simulink library "Mylibrary"  (Simulink 8.3)
settings: Solver=ode45  StartTime=0.0  StopTime=10.0  RelTol=1e-3
undefined symbols (not defined in the file or in its folder): Delay, epsilon, L, Mode, R, T_Trigger, tau_bar, Ts, Ts1, vd, Vehicle_Index, vp, x0, y0
undefined symbols (not defined in the file): d1, m1, psi20, Vx, Vy, x20, y20
libraries: Mylibrary x3
(part 2 of 3)

== matlab function Virtual Target Lapier/Virtual Target Position 2 ==
  settings: updateMethod=DISCRETE  sampleTime=0.2
  data: gamma_c output double; gamma input double size=1; pd output double; vd_bar output double size=1; theta_c output double size=1; vd input double; L input double; R input double; d input double; m input double
function [gamma_c,pd,vd_bar,theta_c] = fcn(gamma,vd,L,R,d,m) 
s1=L-m;
s2=s1+pi*(R-d);
s3=s2+L;
s4=s3+pi*(R+d);
s5=s4+m;
ratio1=(R-d)/R;
ratio2=(R+d)/R;
ratio1=1;
ratio2=1;
if gamma<s5;
    cycle=0;
else
    cycle=1;
end

s=gamma-s5*cycle;

if s<s1                                    % first segment of straight line;
    vd_bar=vd;
    xd=0+d;
    yd=s+R+m;
    theta_c=90;
    gamma_c=s+s5*cycle;                                  % the segment is parallel with x
elseif (s>=s1) && (s<=s2)                  % second segment, a circumference 
    vd_bar=ratio1*vd;
    theta_c=90-(s-s1)*180/((R-d)*pi);
    xd=d+(R-d)*(1-sind(theta_c));
    yd=L+R+(R-d)*cosd(theta_c);   
    gamma_c=s1+(s-s1)*R/(R-d)+s5*cycle; 
elseif (s>s2) && (s<=s3)                   % third segment, a straight line 
    vd_bar=vd;
    yd=s3-s+R;  
    theta_c=-90;
    xd=d+2*(R-d);
    gamma_c=s+d*pi+s5*cycle;
elseif (s>s3) && (s<=s4)   
    vd_bar=ratio2*vd;
    theta_c=-90+(s-s3)/(R+d);
    xd=d+2*(R-d)+(R+d)*(1+sin(theta_c));
    yd=R-(R+d)*cos(theta_c);
    gamma_c=s3+d*pi+(s-s3)*R/(R+d)+s5*cycle;   
else
    vd_bar=vd;
    yd=(s-s4)+R;
    xd=d+4*R;
    theta_c=90;
    gamma_c=s+s5*cycle;
end

if cycle ==0
pd=[xd;cycle*4*R+yd];    
else 
pd=[xd;cycle*4*R+yd];
end

== matlab function Simplified Estimator of Gamma for two vehicle/Estimator ==
  data: vd_t output double size=1; DataToTran output double size=2; gamma_c input double; gamma_c_M input double; t input double; Re_Data1 input double size=2; Re_Data2 input double; Com_Sig input double; gamma_hat output double; tau_bar input double; Mode input double; vd input double; e_int input double; e output double; e_int_event output double
function [vd_t,DataToTran,gamma_hat,e,e_int_event] = fcn(gamma_c,gamma_c_M,t,Re_Data1,Re_Data2,Com_Sig,tau_bar,Mode,vd,e_int)

%% 
kg=1;
% L=[1 -1;
%    -1 1]; 

%% Reset estimator of gamma
persistent gamma_cn1 gamma_cn2 gamma_c0 tc1 tc2 tcn11 tcn12 tcn21 tcn22 tem_c tem_cn1 tem_cn2 reset_c reset_cn1 reset_cn2 e_int_t;   
if isempty(gamma_cn1)
    gamma_cn1=0;
    gamma_cn2=0;
    gamma_c0=0;
    tcn11=t;
    tcn12=t;
    tcn21=t;
    tcn22=t;
    tc1=t;
    tc2=t;
    tem_c=t;
    tem_cn1=t;
    tem_cn2=t;
    reset_c=false;
    reset_cn1=false;
    reset_cn2=false;
    e_int_t=0;
end
%% Reset estimator for gamma_c of first neighbor;
if (Re_Data1(1)~=0)                                  % If recived new data, reset estimator that the current vehicle thinks about the neighbor vehicle
    tcn11=Re_Data1(1); 
    tem_cn1=Re_Data1(2);
    reset_cn1=true;
end   
if (t-tcn11>tau_bar)&&reset_cn1
    gamma_cn1=tem_cn1+vd*tau_bar;
    reset_cn1=false;
    tcn12=t;
end
%% Reset estimator for gamma_c of second neighbor;
if (Re_Data2(1)~=0)                                  % If recived new data, reset estimator that the current vehicle thinks about the neighbor vehicle
    tcn21=Re_Data1(1); 
    tem_cn2=Re_Data2(2);
    reset_cn2=true;
end   
if (t-tcn21>tau_bar)&&reset_cn2
    gamma_cn2=tem_cn2+vd*tau_bar;
    reset_cn2=false;
    tcn22=t;
end
%% Reset estimator for gamma_c of current vehicle   % When it sends its coordinate state to neighbor, it needs to update its estimator too to synchoronize with the neighbor
if (Com_Sig~=0)
    tc1=t;
    tem_c=gamma_c;
    reset_c=true;
end
if (t-tc1>tau_bar)&& reset_c
    gamma_c0=tem_c+vd*tau_bar;
    reset_c=false;
    tc2=t;
end
%% Run estimators
gamma_c_hat=gamma_c0+vd*(t-tc2);
gamma_c_n1_hat=gamma_cn1+vd*(t-tcn12);
gamma_c_n2_hat=gamma_cn2+vd*(t-tcn22);

gamma_hat=[gamma_c_hat;gamma_c_n1_hat;gamma_c_n2_hat]; 

ki=.1;
if Mode==0
     e=gamma_c_M-0.5*(Re_Data1(2)+Re_Data2(2));
elseif Mode==1
    if (Re_Data1(2)~=0)
       e=gamma_c_M-0.5*(Re_Data1(2)+Re_Data2(2));
    else   
       e=0;
    end
else
    if (Re_Data1(2)~=0) 
       e=gamma_c_M-Re_Data1(2);
       e_int_t=e_int_t+e;
    else
        e=0;
    end
     if (Re_Data2(2)~=0) 
       e=gamma_c_M-Re_Data2(2);
       e_int_t=e_int_t+e;
     else
         e=0;
     end
end
%% Compute correction term 
if Mode==0;                                     % if Mode==0, continous communication, we use direct data recieved from neighbor.
    vd_t=-kg*e-ki*e_int; 
elseif Mode==1
    e1=(gamma_c-0.5*(gamma_c_n1_hat+gamma_c_n2_hat));
    vd_t=-kg*e1-ki*e_int;
else
    e1=(gamma_c-0.5*(gamma_c_n1_hat+gamma_c_n2_hat));
    vd_t=-kg*e1-ki*e_int_t;
end
e_int_event=e_int_t;
%% Prepare Data for transmition block
gamma_e=gamma_c-gamma_c_hat;
% DataToTran=[gamma_c;gamma_e;gamma_hat];
DataToTran=[gamma_c;gamma_e];

== matlab function Medusa_Model/State Derivatives ==
  data: x input double; y input double; yaw input double; u input double; v input double; r input double; tau_u input double; dot_x output double; tau_r input double; dot_y output double; dot_yaw output double; dot_u output double; dot_v output double; dot_r output double; fu input double; fv input double; fr input double; Vcx input double; Vcy input double
function [dot_x,dot_y,dot_yaw,dot_u,dot_v,dot_r] = fcn(x,y,yaw,u,v,r,tau_u,tau_r,fu,fv,fr, Vcx, Vcy)
% This is model of Sirene given in the thesis of Vanni

mass = 17.0;
I_z = 1;
X_dot_u = -20;
Y_dot_v = -30;%-1.3175;
N_dot_r = -8.69;% -0.5;
X_u = -0.2;
Y_v = -50;
N_r = -4.14; %-0.1
X_uu = -25; 
Y_vv = -0.01;%-101.2776;
N_rr = -6.23; %-21

%%%%%% masses
m_u = mass - X_dot_u;
m_v = mass - Y_dot_v;
m_r = I_z - N_dot_r;
m_uv = m_u - m_v;

%%%%%%%%% drag

d_u = -X_u - X_uu*abs(u);
d_v = -Y_v - Y_vv*abs(v);
d_r = -N_r - N_rr*abs(r);

%%%%%%%%% Dynamics

dot_u = 1/m_u*(tau_u + m_v*v*r - d_u*u+fu);
dot_v = 1/m_v*(-m_u*u*r - d_v*v+fv);
dot_r = 1/m_r*(tau_r + m_uv*u*v - d_r*r+fr);

dot_x = u*cos(yaw) - v*sin(yaw) + Vcx;
dot_y = u*sin(yaw) + v*cos(yaw) + Vcy;
dot_yaw = r;

== matlab function PF Controller+Medusa/Path Following Controller/Inner-loop controller ==
  settings: sampleTime=Ts
  data: ud_dot input double; ud input double size=2; ur input double; r input double; tau_r output double; tau_u output double; vr_hat input double
function [tau_r,tau_u]  = fcn(ud_dot,ud,ur,r,vr_hat)
%#codegen                        % design speed profile
u=[ur;r];
% Vcxy=[0;0];                       % without constant current in inertial frame
% Vc_hat=R'*Vcxy; 


mass = 17.0;
I_z = 1;
X_dot_u = -20;
Y_dot_v = -30;%-1.3175;
N_dot_r = -8.69;% -0.5;
X_u = -0.2;
N_r = -4.14; %-0.1
X_uu = -25; 
N_rr = -6.23; %-21


dur = -X_u - X_uu*abs(ur);
dr = -N_r - N_rr*abs(r);
D=[dur 0;
    0  dr];

m_u = mass - X_dot_u;
m_v = mass - Y_dot_v;

mr = I_z - N_dot_r;


muv=m_u-m_v;
C=[0 -m_v*vr_hat;
    -muv*vr_hat 0];
M=[m_u 0;
    0 mr];

%% Innerloop controller
    ku=100;kr=10;
    Kd=[ku 0; 
        0 kr];
%     ud_dot=[0;0];
    tau=-Kd*(u-ud)+D*ud+C*u+M*ud_dot;
%% Apply torque and force to vehicles
    tau_u=tau(1);
    tau_r=tau(2);

== matlab function PF Controller+Medusa/Path Following Controller/Observer/observer of current and vr  ==
  settings: sampleTime=Ts
  data: vr_hat_old input double; ur input double; psi input double; p input double size=2; Vcxy_hat_old input double; p_hat_old input double; vr_hat output double; Vc_hat output double; Vcxy_hat output double; p_hat output double; r input double
function [vr_hat,Vc_hat,Vcxy_hat,p_hat]  = Current_obs(vr_hat_old,ur,psi,p,Vcxy_hat_old,p_hat_old,r)
Ts=0.2;
R=[cos(psi)   -sin(psi);
   sin(psi)    cos(psi)]; 
p_t=p-p_hat_old;
Vr=[ur;vr_hat_old];

%% current observer

Kp=10*[1 0;
       0 1];
Kc=10*[1 0;
      0 1];
p_hat=p_hat_old+Ts*(R*Vr+Vcxy_hat_old+Kp*p_t);
Vcxy_hat=Vcxy_hat_old+Ts*Kc*p_t;
%% estimation of vr
mass = 17.0;

X_dot_u = -20;
Y_dot_v = -30;%-1.3175;


Y_v = -50;

Y_vv = -0.01;%-101.2776;
  
  m_u = mass - X_dot_u;
  m_v = mass - Y_dot_v;
  d_v = -Y_v - Y_vv*abs(vr_hat_old);
  
  vr_hat=vr_hat_old+Ts*(-m_u*ur*r/m_v-d_v*vr_hat_old/m_v);
%% Transform the coodinates of current to body frame
Vc_hat=R'*Vcxy_hat;

== matlab function gamma estimator single neighbor/Estimator ==
  data: t input double; Re_Data input double; gamma_dot output double; gamma_c input double; trigger output double; x0 output double; tau_bar input double; Vehicle_Index input double; gamma_hat input double size=2; vd_t output double; DataToTran output double size=4; Mode input double; Com_Sig input double
function [gamma_dot,trigger,x0,vd_t,DataToTran] = fcn(t,Re_Data,gamma_c,tau_bar,Vehicle_Index,gamma_hat,Mode,Com_Sig)

%% compute error term of velocity 
% kg=0.3;
vd=1;kg=0.05;
L=[1 -1;
   -1 1]; 
% trigger=Re_Data(2); 
% x0=[gamma_c;Re_Data(2)];
% gamma_dot = vd*[1;1];

%% Reset estimator of gamma
persistent data_old t_recieve trigger_tem gamma_n;   
if isempty(data_old)
    data_old=Re_Data(1);
    t_recieve=t;
    trigger_tem=0;
    gamma_n=0;
end
if (Re_Data(1)~=0)
    t_recieve=Re_Data(1);
    trigger_tem=0;
    gamma_n=Re_Data(2)+vd*tau_bar;
end 
if (t-t_recieve>tau_bar)
    trigger_tem=1;
end
data_old=Re_Data(1);


x0=[gamma_c;gamma_n];
trigger=trigger_tem;
% gamma_dot = vd*[1;1]-kg*L*gamma_hat;
gamma_dot = vd*[1;1];

%% Compute correction term 
if Mode==0;
    gamma_c_n_hat=Re_Data(2);
else
    gamma_c_n_hat=gamma_hat(2);
end
% gamma_c_hat=gamma_hat(Vehicle_Index);
vd_t=-kg*(gamma_c-gamma_c_n_hat);  
%% Prepare Data for transmition block
gamma_e=gamma_c-gamma_hat(1);
DataToTran=[gamma_c;gamma_e;gamma_hat];

== matlab function PF Controller+Medusa/Path Following Controller/Outer-loop controller ==
  settings: updateMethod=CONTINUOUS  sampleTime=Ts
  data: gamma_dot input double size=1; gamma_ddot output double size=1; pd input double size=2; pd_gamma input double size=2; vd_bar input double; p input double size=2; psi input double; Vc_hat input double size=2; ud output double size=2; vr_hat input double; vd_t input double
function [gamma_ddot,ud]  = fcn(gamma_dot,pd,pd_gamma,vd_bar,p,psi,Vc_hat,vr_hat,vd_t)
%#codegen                        % design speed profile
vd=vd_bar+vd_t;
%% put constraint for vd

%%
R=[cos(psi)   -sin(psi);
   sin(psi)    cos(psi)]; 
e=R'*(p-pd);
% Vcxy=[0;0];                       % without constant current in inertial frame
% Vc_hat=R'*Vcxy; 
%% Outerloop controller
    delta=-0.2;
    Delta_inv= [1    0;
                0 -1/delta]; 
    %     kx=1; ky=0.6;    
    kx=1; ky=0.6;   
    Kk=[kx 0;
        0  ky];
    ud=Delta_inv*(-Kk*tanh(e-[delta;0])-[0;vr_hat]-Vc_hat+R'*pd_gamma*vd);
    
    %
% ud_max=1.5;
% ud_min=-1;
%     
% if ud(1)>=ud_max
%     ud(1)=ud_max;
% elseif ud(1)<=ud_min
%     ud(1)=ud_min;
% end
       
 %% control gamma   
%     kz=100;
    kz=30;
    vd_dot=0;
    gamma_ddot=-kz*(gamma_dot-vd_bar)+vd_dot+(e-[delta;0])'*R'*pd_gamma + kz*vd_t;  % not that, vd=constant => vd_partial=0 => z=gamma_dot
    %gamma_ddot=0;

== matlab function  Real MEDUSA Vehicle (2013)/Medusa/Dynamics1/State Derivatives ==
  data: x input double; y input double; yaw input double; u input double; v input double; r input double; tau_u input double; dot_x output double; tau_r input double; dot_y output double; dot_yaw output double; dot_u output double; dot_v output double; dot_r output double; fu input double; fv input double; fr input double; Vcx input double; Vcy input double
function [dot_x,dot_y,dot_yaw,dot_u,dot_v,dot_r] = fcn(x,y,yaw,u,v,r,tau_u,tau_r,fu,fv,fr, Vcx, Vcy)
%state = [x, y, yaw, u, v, r]

% %%%%%% Coefficients
% mass = 17.0;
% I_z = 4.14;
% X_dot_u = -20;
% Y_dot_v = -1.3175;
% N_dot_r =  -8.69;
% X_u = -0.2;
% Y_v = -55.117;
% N_r = -4.14;
% X_uu = -25; 
% Y_vv = -101.2776;
% N_rr = -6.23;

%%%%%% Coefficients
mass = 17.0;
I_z = 1;
X_dot_u = -20;
Y_dot_v = -30;%-1.3175;
N_dot_r = -8.69;% -0.5;
X_u = -0.2;
Y_v = -50;
N_r = -4.14; %-0.1
X_uu = -25; 
Y_vv = -0.01;%-101.2776;
N_rr = -6.23; %-21

%%%%%% masses
m_u = mass - X_dot_u;
m_v = mass - Y_dot_v;
m_r = I_z - N_dot_r;
m_uv = m_u - m_v;

%%%%%%%%% drag

d_u = -X_u - X_uu*abs(u);
d_v = -Y_v - Y_vv*abs(v);
d_r = -N_r - N_rr*abs(r);

%%%%%%%%% Dynamics

dot_u = 1/m_u*(tau_u + m_v*v*r - d_u*u+fu);
dot_v = 1/m_v*(-m_u*u*r - d_v*v+fv);
dot_r = 1/m_r*(tau_r + m_uv*u*v - d_r*r+fr);

dot_x = u*cos(yaw) - v*sin(yaw) + Vcx;
dot_y = u*sin(yaw) + v*cos(yaw) + Vcy;
dot_yaw = r;

== matlab function  Real MEDUSA Vehicle (2013)/Medusa/Heading Controller/Embedded MATLAB Function1 ==
  data: YawRef input double; x output double; Yaw input double; Yawrate input double; Kd parameter double; Kp parameter double
function x = controller(YawRef, Yaw, Yawrate, Kd, Kp)
err = ( YawRef- Yaw );
if(err>180) 
     err=err-360;
elseif(err<-180) 
     err=360+err;
end

x=Kp*err-Kd*Yawrate;

== matlab function  Real MEDUSA Vehicle (2013)/Medusa/MotorPower/Embedded MATLAB Function ==
  data: Sm output double; Pm output double; Cm_Speed input double; Dm_Head input double; Cm input double; Dm input double; InnerLoops input double
function [Sm,Pm] = fcn(Cm_Speed, Dm_Head, Cm, Dm, InnerLoops)
Cm_sqr=0;
Dm_sqr=0;
% switch InnerLoops
%     case 0
%         ; % Don't do anything
%     case 1
%         Cm_sqr=Cm_Speed;
%         Dm_sqr=Dm_Head;
%     case 2
%         Cm_sqr=Cm*abs(Cm);
%         Dm_sqr=Dm_Head;
%     case 3
%         Cm_sqr=Cm_Speed;
%         Dm_sqr=Dm*abs(Dm);
%     case 4
        Cm_sqr=Cm*abs(Cm);
        Dm_sqr=Dm*abs(Dm);
%     otherwise
% end

Pm = round(sqrt(abs(Cm_sqr+Dm_sqr))*sign(Cm_sqr+Dm_sqr));
Sm = round(sqrt(abs(Cm_sqr-Dm_sqr))*sign(Cm_sqr-Dm_sqr));

== matlab function PF Controller Lapier Miguel Hung  ==
  settings: updateMethod=DISCRETE  sampleTime=0.2
  data: vd_t input double size=1; p input double size=2; r input double; yaw input double size=1; u input double size=1; gamma_c output double size=1; vcxy_hat output double; yaw_ref output double; r_ref output double; precise output double; u_ref output double; pd output double; L parameter double; R parameter double; d parameter double; m parameter double; vd parameter double
function [gamma_c,vcxy_hat,yaw_ref,r_ref,precise,u_ref,pd] = fcn(vd_t,p,r,yaw,u,L, R, d, m, vd)
%% Declare and initialize global variales                                   These variables will be kept in memory during execuation
    Ts=0.2;         
    persistent vr_hat_old   vr_hat    % sampling time
    persistent p_hat_old    p_hat   Vcxy_hat_old Vcxy_hat 
    persistent gamma_old gamma_dot_old
    if isempty(p_hat)
        vr_hat_old=0;            vr_hat=0; 
        p_hat=p;                 p_hat_old=p;    Vcxy_hat_old=[0;0];  Vcxy_hat=[0;0];
        gamma_old=0;  
        gamma_dot_old=0;
    end    
%% Vehicle Prameters
    mass = 17.0;
    X_dot_u = -20;
    Y_dot_v = -30;                                                              %-1.3175;
    Y_v = -50;
    Y_vv = -0.01;                                                               %-101.2776;
    % masses
    m_u = mass - X_dot_u;
    m_v = mass - Y_dot_v;
    N_r = -4.14; %-0.1
    N_rr = -6.23; %-21
%% Update path
    [gamma_c,vd_bar,path_point,s_dot] = path(gamma_old,L, R, d, m, vd);
    theta_c=path_point(3)*180/pi;
    c_c=path_point(5);
    g_c=path_point(6);
    pd=[path_point(1);path_point(2)];
%% error between vehicle and rabbit
   R1=[cosd(theta_c)       sind(theta_c);     % From {I} to {F}
      -sind(theta_c)       cosd(theta_c)]; 
   e=p-pd;
   e_f=R1*e;
   s1=e_f(1);
   y1=e_f(2);      
%% Estimate vr
    d_v = -Y_v - Y_vv*abs(vr_hat);
    vr_hat_dot=-m_u*u*r/m_v-d_v*vr_hat/m_v;
    vr_hat=vr_hat_old+Ts*vr_hat_dot;
    vr_hat_old=vr_hat; 
%% Estimate current 
% Estimate current in Inertial frame
    R2=[cosd(yaw)        -sind(yaw);     % From {B} to {I}
        sind(yaw)         cosd(yaw)]; 
    p_t=p-p_hat;
    Vr=[u;0*vr_hat];
    Kp=10*[1 0;
           0 1];
    Kc=10*[1 0;
          0 1];
    p_hat_dot=R2*Vr+Vcxy_hat+Kp*p_t;
    p_hat=p_hat_old+Ts*p_hat_dot;
    p_hat_old=p_hat;
    Vcxy_hat_dot=Kc*p_t;
    Vcxy_hat=Vcxy_hat_old+Ts*Vcxy_hat_dot;
    Vcxy_hat_old=Vcxy_hat;
    vcxy_hat=Vcxy_hat;
% Transform the estimated current to Frenet frame
    Vc_hat_f=R1*Vcxy_hat;                      
    Vc_par=Vc_hat_f(1);
    Vc_per=Vc_hat_f(2);
%% Outerloop Controller
   s=2;
   a=y1/s+Vc_per/u;
%    a=y1/s;                                             % No current                          
   a= min(max(a, -1), 1);
   theta=-asind(a);
% Yaw reference
   yaw_ref=theta_c+theta;
%    yaw_ref=60;
% Yaw rate reference
    r_ref=-c_c*s_dot*180/pi;
%     r_ref=0;
% speed reference
    u_ref=vd_bar+vd_t;
%% Gamma Controller
   k1=1;
   gamma_dot=u*cosd(yaw-theta_c)+k1*s1+Vc_par;
   s_acc=(gamma_dot-gamma_dot_old)/Ts;
   gamma_dot_old=gamma_dot;
   gamma=gamma_old+Ts*gamma_dot;
   gamma_old=gamma;
% Precicise 
    r_rad=r*pi/180;
    precise=-g_c*s_dot^2-c_c*s_acc - N_r*r_rad - N_rr*r_rad*abs(r_rad);
%     precise=0;
end
function [gamma_c,vd_bar,path_point,s_dot] = path(gamma,L, R, d, m, vd) 
s1=L-m;
s2=s1+pi*(R-d);
s3=s2+L;
s4=s3+pi*(R+d);
s5=s4+m;
ratio1=(R-d)/R;
ratio2=(R+d)/R;
ratio1=1;
ratio2=1;
if gamma<s5;
    cycle=0;
else
    cycle=1;
end
Ts=0.2;
s=gamma-s5*cycle;

persistent c_c_old gamma_old
if isempty(c_c_old)
    c_c_old=0;
    gamma_old=0;
end

if s<s1                                    % first segment of straight line;
    vd_bar=vd;
    xd=0+d;
    yd=s+R+m;
    theta_c=pi/2;
    gamma_c=s+s5*cycle;                    % the segment is parallel with x
    c_c=0;
    c_c_dot=c_c-c_c_old;
    s_dot=(gamma-gamma_old)/Ts;
    g_c=c_c_dot/s_dot;                                 % g_c=c_c_dot/s_dot;
elseif (s>=s1) && (s<=s2)                  % second segment, a circumference 
    vd_bar=ratio1*vd;
    theta_c=pi/2-(s-s1)/((R-d));
    xd=d+(R-d)*(1-sin(theta_c));
    yd=L+R+(R-d)*cos(theta_c);   
    gamma_c=s1+(s-s1)*R/(R-d)+s5*cycle; 
    c_c=1/(R-d);
    c_c_dot=c_c-c_c_old;
    s_dot=(gamma-gamma_old)/Ts;
    g_c=c_c_dot/s_dot;                                 % g_c=c_c_dot/s_dot;
elseif (s>s2) && (s<=s3)                   % third segment, a straight line 
    vd_bar=vd;
    yd=s3-s+R;  
    theta_c=-pi/2;
    xd=d+2*(R-d);
    gamma_c=s+d*pi+s5*cycle;
    c_c=0;
    c_c_dot=c_c-c_c_old;
    s_dot=(gamma-gamma_old)/Ts;
    g_c=c_c_dot/s_dot;                                 % g_c=c_c_dot/s_dot;
elseif (s>s3) && (s<=s4)   
    vd_bar=ratio2*vd;
    theta_c=-pi/2+(s-s3)/(R+d);
    xd=d+2*(R-d)+(R+d)*(1+sin(theta_c));
    yd=R-(R+d)*cos(theta_c);
    gamma_c=s3+d*pi+(s-s3)*R/(R+d)+s5*cycle;   
    c_c=-1/(R+d);
    c_c_dot=c_c-c_c_old;
    s_dot=(gamma-gamma_old)/Ts;
    g_c=c_c_dot/s_dot;                                 % g_c=c_c_dot/s_dot;
else
    vd_bar=vd;
    yd=(s-s4)+R;
    xd=d+4*R;
    theta_c=pi;
    gamma_c=s+s5*cycle;
    c_c=0;
    c_c_dot=c_c-c_c_old;
    s_dot=(gamma-gamma_old)/Ts;
    g_c=c_c_dot/s_dot;                                 % g_c=c_c_dot/s_dot;
end
if s_dot==0
    g_c=0;
else
    g_c=c_c_dot/s_dot; 
end   
c_c_old=c_c;
gamma_old=gamma;
path_point=[cycle*4*R+xd,yd,theta_c, gamma,c_c,g_c];
end

== matlab function Real Medusa/Dynamics1/State Derivatives ==
  data: x input double; y input double; yaw input double; u input double; v input double; r input double; tau_u input double; dot_x output double; tau_r input double; dot_y output double; dot_yaw output double; dot_u output double; dot_v output double; dot_r output double; fu input double; fv input double; fr input double; Vcx input double; Vcy input double
function [dot_x,dot_y,dot_yaw,dot_u,dot_v,dot_r] = fcn(x,y,yaw,u,v,r,tau_u,tau_r,fu,fv,fr, Vcx, Vcy)
%state = [x, y, yaw, u, v, r]

% %%%%%% Coefficients
% mass = 17.0;
% I_z = 4.14;
% X_dot_u = -20;
% Y_dot_v = -1.3175;
% N_dot_r =  -8.69;
% X_u = -0.2;
% Y_v = -55.117;
% N_r = -4.14;
% X_uu = -25; 
% Y_vv = -101.2776;
% N_rr = -6.23;

%%%%%% Coefficients
mass = 17.0;
I_z = 1;
X_dot_u = -20;
Y_dot_v = -30;%-1.3175;
N_dot_r = -8.69;% -0.5;
X_u = -0.2;
Y_v = -50;
N_r = -4.14; %-0.1
X_uu = -25; 
Y_vv = -0.01;%-101.2776;
N_rr = -6.23; %-21

%%%%%% masses
m_u = mass - X_dot_u;
m_v = mass - Y_dot_v;
m_r = I_z - N_dot_r;
m_uv = m_u - m_v;

%%%%%%%%% drag

d_u = -X_u - X_uu*abs(u);
d_v = -Y_v - Y_vv*abs(v);
d_r = -N_r - N_rr*abs(r);

%%%%%%%%% Dynamics

dot_u = 1/m_u*(tau_u + m_v*v*r - d_u*u+fu);
dot_v = 1/m_v*(-m_u*u*r - d_v*v+fv);
dot_r = 1/m_r*(tau_r + m_uv*u*v - d_r*r+fr);

dot_x = u*cos(yaw) - v*sin(yaw) + Vcx;
dot_y = u*sin(yaw) + v*cos(yaw) + Vcy;
dot_yaw = r;

== matlab function Real Medusa/Heading Controller/Embedded MATLAB Function1 ==
  data: YawRef input double; x output double; Yaw input double; Yawrate input double; Kd parameter double; Kp parameter double
function x = controller(YawRef, Yaw, Yawrate, Kd, Kp)
err = ( YawRef- Yaw );
if(err>180) 
     err=err-360;
elseif(err<-180) 
     err=360+err;
end

x=Kp*err-Kd*Yawrate;

== matlab function Real Medusa/MotorPower/Embedded MATLAB Function ==
  data: Sm output double; Pm output double; Cm_Speed input double; Dm_Head input double; Cm input double; Dm input double; InnerLoops input double
function [Sm,Pm] = fcn(Cm_Speed, Dm_Head, Cm, Dm, InnerLoops)
Cm_sqr=0;
Dm_sqr=0;
switch InnerLoops
    case 0
        ; % Don't do anything
    case 1
        Cm_sqr=Cm_Speed;
        Dm_sqr=Dm_Head;
    case 2
        Cm_sqr=Cm*abs(Cm);
        Dm_sqr=Dm_Head;
    case 3
        Cm_sqr=Cm_Speed;
        Dm_sqr=Dm*abs(Dm);
    case 4
        Cm_sqr=Cm*abs(Cm);
        Dm_sqr=Dm*abs(Dm);
    otherwise
end

Pm = round(sqrt(abs(Cm_sqr+Dm_sqr))*sign(Cm_sqr+Dm_sqr));
Sm = round(sqrt(abs(Cm_sqr-Dm_sqr))*sign(Cm_sqr-Dm_sqr));

== matlab function PF Controller Vanni  ==
  settings: updateMethod=DISCRETE  sampleTime=0.2
  data: pd input double; pd_gamma input double; vd_bar input double; vd_t input double size=1; r input double size=1; u input double size=1; yaw input double size=1; p input double size=2; gamma output double size=1; vcxy_hat output double; u_d output double; r_d output double; vd output double; tau_u output double; tau_r output double; m output double; K output double; ky output double
function [gamma,vcxy_hat,u_d,r_d,vd,tau_u,tau_r,m,K,ky] = fcn(pd,pd_gamma,vd_bar,vd_t,r,u,yaw,p)

%% Vehicle parameters
% 
%     mass = 17.0;
%     I_z = 1;
%     X_dot_u = -20;
%     Y_dot_v = -30;                                                              %-1.3175;
%     N_dot_r = -8.69;                                                            % -0.5;
%     X_u = -0.2;
%     Y_v = -50;
%     N_r = -4.14;                                                                %-0.1
%     X_uu = -25; 
%     Y_vv = -0.01;                                                               %-101.2776;
%     N_rr = -6.23;                                                               %-21
% 
%     % masses
%     m_u = mass - X_dot_u;
%     m_v = mass - Y_dot_v;
%     mr = I_z - N_dot_r;
%     muv=m_u-m_v;
%    
% % drag
%     du = -X_u - X_uu*abs(u);
%     dr = -N_r - N_rr*abs(r);

%% Declare and initialize global variales                                   These variables will be kept in memory during execuation

   
    persistent vr_hat_old   vr_hat                                              % to estimate vr
    persistent p_hat_old    p_hat   Vcxy_hat_old Vcxy_hat 
    persistent gamma_dot_old gamma_dot gamma_old
    persistent ud_old ud_t
    persistent eu_int
    persistent eu_old tau_u_old
    persistent er_old tau_r_old
    persistent ed_int
    persistent vd_bar_old vd_bar_out
    persistent vd_old vd_new
    persistent lock

    if isempty(vr_hat)
        vr_hat_old=0;           vr_hat=0; 
        p_hat=p;                p_hat_old=p;    Vcxy_hat_old=[0;0];  Vcxy_hat=[0;0];
        gamma_dot_old=0;        gamma_dot=0;    gamma_old=0;
        ud_old=[0;0];           ud_t=[0;0]
        eu_int=[0;0];
        eu_old=0; tau_u_old=0;
        er_old=0; tau_r_old=0;
        ed_int=[0;0];
        vd_bar_old=0;
        vd_bar_out=0;
        vd_old=0; vd_new=0;
        lock=1;
    end
%%  Smooth vd_bar
Ts=0.2;                                                                     % sampling time
% time_c=5;   % five second smooth
% a=1/time_c;
% vd_bar_out=a*vd_bar+exp(-a*Ts)*vd_bar_old;
% vd_bar_old=vd_bar_out;
vd=vd_bar+vd_t;
vd_new=vd;    
%% Calculate rotation matrix
  
    R=[cosd(yaw)   -sind(yaw);
       sind(yaw)    cosd(yaw)]; 
%% Estimate vr

%     d_v = -Y_v - Y_vv*abs(vr_hat);
%     vr_hat_dot=-m_u*u*r/m_v-d_v*vr_hat/m_v;
%     vr_hat=vr_hat_old+Ts*vr_hat_dot;
%     vr_hat_old=vr_hat;
%     vr_hat_out=vr_hat;
%% Estimate current 

% Estimate current in Inertial frame

    p_t=p-p_hat;
    Vr=[u;0];
    Kp=10*[1 0;
           0 1];
    Kc=10*[1 0;
          0 1];
    p_hat_dot=R*Vr+Vcxy_hat+Kp*p_t;
    p_hat=p_hat_old+Ts*p_hat_dot;
    p_hat_old=p_hat;
    Vcxy_hat_dot=Kc*p_t;
    Vcxy_hat=Vcxy_hat_old+Ts*Vcxy_hat_dot;
    Vcxy_hat_old=Vcxy_hat;
    vcxy_hat=Vcxy_hat;
% Transform the estimated current to Body frame
%     Vcxy_hat=[0.12;0.12];
    Vc_hat=R'*Vcxy_hat;

%% Outerloop Controller
    e_out=R'*(p-pd);
  
    delta=-0.2;
    Delta_inv= 1*[1    0;
                0 -1/delta];     
    if abs(pd_gamma(1))==1
        ky=0.15;
        ky=0.2;
    else
        ky=0.2;
    end
     kx=.3; 
%      ky=.2;   
    Kk=[kx 0;
        0  ky];
    K=norm(e_out);
    if (K>0.5)&&(lock==1)
    vd=vd*(1-K/25);
%     vd=0.2;
    ky=0.2*K+0.1;
    else
    lock=0;
    end
           
%     if mod(t,1*Ts)==0
      ed_int=ed_int+(e_out-[delta;0]);
%       ud_t=Delta_inv*(-Kk*tanh(e_out-[delta;0])- 0*[0;vr_hat]-Vc_hat+R'*pd_gamma*vd);  
      ud_t=Delta_inv*(-Kk*tanh(e_out-[delta;0])-Vc_hat+R'*pd_gamma*vd);  
      ud_dot=ud_t-ud_old;
      ud_old=ud_t;
%     else
%         ud_dot=[0;0];
%     end
%     if abs(pd_gamma(1))==1
%       m=0.02;    %  tuning trick, a
%     else
%       m=0.2;  
%     end
      m=0.1*(1-pd_gamma(1)^8)+0.05;    %  tuning trick, a
      ud=[1 0; 0 m]*ud_t;
%       ud=[0.5;0.3];
      u_d=ud(1);
%       r_d=ud(2); 
      r_d=ud(2)*360/(2*pi); 
%% Inner Loop Controller
%  Noted that Inner loop controller use Vanni Vanni method (it does not work well
%  since the model now is not valid because of including of thruster part
%%%%%%%%%%%%%%%%%%%%%%%%%%%%%%%%%%%%%%%%%%%%%%%%%%%%%%%%%%%%%%%%%%%%%%%%%%%%%%%%%%
%     ur=[u;r];
%     C=[ 0            -m_v*vr_hat;
%         -muv*vr_hat            0];
%     M=[ m_u      0;
%         0       mr];
%     D=[ du      0;
%         0       dr];
%     ku=10;kr=10;
%     Kd=[ku 0; 
%         0 kr];
%     Ki=0.01*Kd;   
%     e=ur-ud;
%     eu_int=eu_int+e;
%     tau=-Kd*(ur-ud)+D*ud+C*ur+M*ud_dot-Ki*eu_int;
%     Amplify the tau_u, tau_r to compesate the dynamics of thrusters 
%     tau_u=tau(1)/0.36;
%     tau_r=tau(2)/0.09;
%%%%%%%%%%%%%%%%%%%%%%%%%%%%%%%%%%%%%%%%%%%%%%%%%%%%%%%%%%%%%%%%%%%%%%%%%%%%%%%%%%   
% We can use PID controllers to track ud in innerloop, but this PID is not
% good enough, the better one is the one design outside of this 
 
eu=u_d-u;
er=r_d-r ;
Kp_u=30;
KI_u=10;
KD_u=0;

tau_u=Kp_u*eu+(Ts*KI_u-Kp_u)*eu_old+tau_u_old;
tau_u_old=tau_u;
eu_old=eu;

Kp_r=10;
KI_r=2;
KD_r=0;
% if (psi_T~=0)&&(psi_T~=180)
%     K_yaw=0.000;
% else
%     K_yaw=0;
% end
% if (180<yaw)||(yaw<360)
%     e_yaw=psi_T-(yaw-360);
% else
%     e_yaw=psi_T-yaw;
% end
% tau_r=Kp_r*er+(Ts*KI_r-Kp_r)*er_old+tau_r_old+K_yaw*e_yaw;
tau_r=Kp_r*er+(Ts*KI_r-Kp_r)*er_old+tau_r_old;
tau_r_old=tau_r;
er_old=er;

%% Gamma Controller
    kz=1;
    vd_dot=(vd_new-vd_old)/Ts;   % constant speed profile 
    vd_old=vd_new;
    gamma_ddot=-kz*(gamma_dot-vd_bar)+vd_dot+2*(e_out-[delta;0])'*R'*pd_gamma + kz*vd_t; 
    gamma_dot=gamma_dot_old+Ts*gamma_ddot;
    gamma=gamma_old+Ts*gamma_dot;
    gamma_dot_old=gamma_dot;
    gamma_old=gamma;
end

== matlab function Real Medusa/Speed Controller /Embedded MATLAB Function1 ==
  data: Cm output double; Uref input double; Kpu parameter double; Kiu parameter double; qsiold input double; qsi output double; Vx input double; Vy input double; yaw input double; u output double; us input double; KSat parameter double
function [Cm, qsi, u] = controller(Uref, Kpu,Kiu, qsiold,Vx,Vy,yaw, us, KSat)
u=Vx*sind(yaw)+Vy*cosd(yaw);
err=u-Uref;
qsi=qsiold+err;

Cm=-Kpu*(err+us)-Kiu*qsi;
% Cm =+40*Uref-Kiu*qsi;
% if(t>10)
%     qsi=qsiold+err;
%     Cm =-Kpu*err-Kiu*qsi;
% end
if(abs(Cm) >= KSat)
   Cm = KSat*sign(Cm); 
   qsi = qsiold;
end

== matlab function Virtual Target/Virtual Target Position 2 ==
  settings: updateMethod=DISCRETE  sampleTime=0.2
  data: gamma_c output double; gamma input double size=1; pd output double; pd_gamma output double size=2; vd_bar output double size=1; vd input double; L input double; R input double; d input double; m input double; psi_T output double
function [gamma_c,pd,pd_gamma,vd_bar,psi_T] = fcn(gamma,vd,L,R,d,m) 
s1=L-m;
s2=s1+pi*(R-d);
s3=s2+L;
s4=s3+pi*(R+d);
s5=s4+m;
ratio1=(R-d)/R;
ratio2=(R+d)/R;
% ratio1=1;
% ratio2=1;
delta=0;
v_min=vd;
if gamma<s5;
    cycle=0;
else
    cycle=1;
end

s=gamma-s5*cycle;

if s<s1                                    % first segment of straight line;
    if s1-s<=delta
      vd_bar=v_min+(vd-v_min)*(s1-s)^2/delta^2;
    elseif s<=delta
        if cycle>=1
        vd_bar=v_min+(vd-v_min)*s^2/delta^2;
        else
        vd_bar=vd;
        end
    else
     vd_bar=vd; 
    end
%     vd_bar=vd;
    xd=s+R+m;
    yd=0+d;
    pd_gamma=[1;0];      
    gamma_c=s+s5*cycle;                                  % the segment is parallel with x
    psi_T=0;
elseif (s>=s1) && (s<=s2)                  % second segment, a circumference 
    if (s-s1)<=delta
    vd_bar=v_min+(ratio1*vd-v_min)*(s-s1)^2/delta^2;
    elseif (s2-s)<=delta
    vd_bar=v_min+(ratio1*vd-v_min)*(s2-s)^2/delta^2;   
    else
    vd_bar=ratio1*vd;
    end  
    psi_T=(s-s1)/(R-d);
    xd=L+R+(R-d)*sin(psi_T);   
    yd=d+(R-d)*(1-cos(psi_T));
    pd_gamma=[cos(psi_T);sin(psi_T)];
    gamma_c=s1+(s-s1)*R/(R-d)+s5*cycle; 
    psi_T=psi_T*180/pi;
elseif (s>s2) && (s<=s3)                   % third segment, a straight line 
    if (s-s2)<=delta
    vd_bar=v_min+(vd-v_min)*(s-s2)^2/delta^2;
    elseif (s3-s)<=delta
    vd_bar=v_min+(vd-v_min)*(s3-s)^2/delta^2;    
    else
    vd_bar=vd;
    end
%     vd_bar=vd_bar;
    xd=s3-s+R;  
    yd=d+2*(R-d); 
    pd_gamma=[-1;0];
    gamma_c=s+d*pi+s5*cycle;
    psi_T=180;
elseif (s>s3) && (s<=s4)   
    if (s-s3)<=delta
    vd_bar=v_min+(ratio2*vd-v_min)*(s-s3)^2/delta^2;
    elseif (s4-s)<=delta
    vd_bar=v_min+(ratio2*vd-v_min)*(s4-s)^2/delta^2;    
    else
    vd_bar=ratio2*vd;
    end
    xd=R-(R+d)*sin((s-s3)/(R+d));
    yd=d+2*(R-d)+(R+d)*(1-cos((s-s3)/(R+d)));
    pd_gamma=[-cos((s-s3)/(R+d));sin((s-s3)/(R+d))]; 
    gamma_c=s3+d*pi+(s-s3)*R/(R+d)+s5*cycle;   
    psi_T=180-180*(s-s3)/(R+d)/pi;
else
    if s-s4>=delta
    vd_bar=vd;
    else
    vd_bar=v_min+(vd-v_min)*(s-s4)^2/delta^2;
    end
    vd_bar=ratio1*vd_bar;
    xd=(s-s4)+R;
    yd=d+4*R;
    pd_gamma=[1;0];
    gamma_c=s+s5*cycle;
    psi_T=0;
end

if cycle ==0
pd=[xd;cycle*4*R+yd];
else 
pd=[xd;cycle*4*R+yd];
end

== matlab function CPF Controller Latest version   ==
  settings: updateMethod=DISCRETE  sampleTime=0.2
  data: t input double size=1; Re_Data1 input double size=2; Re_Data2 input double size=2; Com_Sig input double size=1; u input double size=1; r input double size=1; yaw input double size=1; p input double size=2; L parameter double; R parameter double; d parameter double; m parameter double; u_d output double; r_d output double; Com_Mode output double size=1; Diff_Mode output double size=1; DataToTran output double size=2; vd_t output double; tau_bar parameter double size=1; vp parameter double size=1; pd output double
%% CPF is Event/Time Trigger Coordinated Pathfollowing
function [u_d,r_d,Com_Mode,Diff_Mode,DataToTran,vd_t,pd] = CPF(t,Re_Data1,Re_Data2,Com_Sig,u,r,yaw,p,L, R, d, m,tau_bar, vp)
%% Declare variables
persistent  gamma gamma_c_M 
if isempty (gamma)
         gamma=0; gamma_c_M=0;                                              % Noted that we can start any value of gamma here
end
if t<5                                                                      % Wait for update GPS... I am not sure, must be confirmed by experts            
    Com_Mode=0;Diff_Mode=0;
    DataToTran=[0;0];  
    u_d=0;
    r_d=0;
    vd_t=0;
    pd=[0;0];
else
% Update the path and coordination state gamma_c
    [gamma_c,pd,pd_gamma,vd_bar] = path(gamma,vp,L,R,d,m);
    
%% Calculate correction speed from coordination law
    Ts=0.2;    
    [vd_t,DataToTran] = Coordination(t,gamma_c,gamma_c_M,Re_Data1,Re_Data2,Com_Sig,tau_bar,vp);
%% Implement Path Following Controller
%     vd_t=0;
    [gamma_next,u_d,r_d,Com_Mode,Diff_Mode] = PF(t,pd,pd_gamma,vd_bar,vd_t,u,r,yaw,p,Ts);
    
%% Update
    gamma_c_M=gamma_c;
    gamma=gamma_next;
end
end

%% PF is Path Flollowing Controller                                  
function [gamma_next,u_d,r_d,Com_Mode,Diff_Mode] = PF(t,pd,pd_gamma,vd_bar,vd_t,u,r,yaw,p,Ts)

%% Declare and initialize global variales                                   These variables will be kept in memory during execuation
    persistent p_hat_old    p_hat   Vcxy_hat_old Vcxy_hat 
    persistent gamma_dot_old gamma_dot gamma_old
    persistent ud_t
    persistent eu_old Com_Mode_old
    persistent er_old Diff_Mode_old
    persistent ed_int
    persistent vd_old vd_new
    persistent lock
    
    if isempty(p_hat_old)
        p_hat=p;                p_hat_old=p;    Vcxy_hat_old=[0;0];  Vcxy_hat=[0;0];
        gamma_dot_old=0;        gamma_dot=0;    gamma_old=0;
        eu_old=0; Com_Mode_old=0;
        er_old=0; Diff_Mode_old=0;
        ed_int=[0;0];
        vd_old=0; vd_new=0;
        lock=0;
    end
                                                          
%% Calculate rotation matrix from body frame to inertial frame
  
    R=[cosd(yaw)   -sind(yaw);
       sind(yaw)    cosd(yaw)]; 

%% Estimate current 
% Estimate current in Inertial frame
    p_t=p-p_hat;
    Vr=[u;0];
    Kp=10*[1 0;
           0 1];
    Kc=10*[1 0;
          0 1];
    p_hat_dot=R*Vr+Vcxy_hat+Kp*p_t;
    p_hat=p_hat_old+Ts*p_hat_dot;
    p_hat_old=p_hat;
    Vcxy_hat_dot=Kc*p_t;
    Vcxy_hat=Vcxy_hat_old+Ts*Vcxy_hat_dot;
    Vcxy_hat_old=Vcxy_hat;
% Transform the estimated current to Body frame
    Vc_hat=R'*Vcxy_hat;

%% Outerloop Controller
    vd=vd_bar+vd_t;
    e_out=R'*(p-pd);
    delta=-0.2;
    Delta_inv= 1*[1    0;
                0 -1/delta];     
    kx=.3; 
    K=norm(e_out);
    if (K>0.5)&&(lock==1)
        vd=vd*(1-K/25);
        ky=0.1*(1-K/50);
        ky=0.2;
    else
        lock=0;
        ky=0.2;
    end
      Kk=[kx 0;
        0  ky];
      ed_int=ed_int+(e_out-[delta;0]);
      ud_t=Delta_inv*(-Kk*tanh(e_out-[delta;0])- 0*[0;0]-Vc_hat+R'*pd_gamma*vd);  
      m=0.1*(1-pd_gamma(1)^8)+0.05;    %  tuning trick, a
      n=1;
      if t<100
      m=t*0.0015;
      else
      m=0.15;    
%         m=0.1*(1-pd_gamma(1)^8)+0.05;    %  tuning trick, a
      end
      ud=[n 0; 0 m]*ud_t;
      u_d=ud(1);
      r_d=ud(2)*180/(pi); 
%% Inner Loop Controller
    eu=u_d-u;
    er=r_d-r;
    % Speed controller
    Kp_u=30;
    KI_u=10;
    KD_u=0;
    Com_Mode=Kp_u*eu+(Ts*KI_u-Kp_u)*eu_old+Com_Mode_old;
    Com_Mode_old=Com_Mode;
    eu_old=eu;
    % Yaw rate controller
    Kp_r=10;
    KI_r=2;
    KD_r=0;
    Diff_Mode=Kp_r*er+(Ts*KI_r-Kp_r)*er_old+Diff_Mode_old;
    Diff_Mode_old=Diff_Mode;
    er_old=er;

%% Gamma Controller
    kz=4;
    vd_dot=(vd_new-vd_old)/Ts;   
    vd_old=vd_new;
    gamma_ddot=-kz*(gamma_dot-vd_bar)+vd_dot+2*(e_out-[delta;0])'*R'*pd_gamma + kz*vd_t; 
    gamma_dot=gamma_dot_old+Ts*gamma_ddot;
    gamma_next=gamma_old+Ts*gamma_dot;
    gamma_dot_old=gamma_dot;
    gamma_old=gamma_next;
end                 
%% Coordinaiton is Time/Event Trigger Cordination Law
function [vd_t,DataToTran] = Coordination(t,gamma_c,gamma_c_M,Re_Data1,Re_Data2,Com_Sig,tau_bar,vp)

%% Declare variables
    persistent gamma_cn1 gamma_cn2 gamma_c0 tc1 tc2 tcn11 tcn12 tcn21 tcn22 tem_c tem_cn1 tem_cn2 reset_c reset_cn1 reset_cn2 e_int_t;   
    if isempty(gamma_cn1)
        gamma_cn1=0;gamma_cn2=0;
        gamma_c0=0;
        tcn11=t;tcn12=t;
        tcn21=t;tcn22=t;
        tc1=t;tc2=t;
        tem_c=t;
        tem_cn1=t;tem_cn2=t;
        reset_c=false;
        reset_cn1=false;
        reset_cn2=false;
        e_int_t=0;
    end
%% Reset estimator for gamma_c of first neighbor;
    if (Re_Data1(1)~=0)                                  % If recived new data, reset estimator that the current vehicle thinks about the neighbor vehicle
        tcn11=Re_Data1(1); 
        tem_cn1=Re_Data1(2);
        reset_cn1=true;
    end   
    if (t-tcn11>tau_bar)&&reset_cn1
        gamma_cn1=tem_cn1+vp*tau_bar;
        reset_cn1=false;
        tcn12=t;
    end
%% Reset estimator for gamma_c of second neighbor;
    if (Re_Data2(1)~=0)                                  % If recived new data, reset estimator that the current vehicle thinks about the neighbor vehicle
        tcn21=Re_Data2(1); 
        tem_cn2=Re_Data2(2);
        reset_cn2=true;
    end   
    if (t-tcn21>tau_bar)&&reset_cn2
        gamma_cn2=tem_cn2+vp*tau_bar;
        reset_cn2=false;
        tcn22=t;
    end
%% Reset estimator for gamma_c of current vehicle   % When it sends its coordinate state to neighbor, it needs to update its estimator too to synchoronize with the neighbor
    if (Com_Sig~=0)
        tc1=t;
        tem_c=gamma_c;
        reset_c=true;
    end
    if (t-tc1>tau_bar)&& reset_c
        gamma_c0=tem_c+vp*tau_bar;
        reset_c=false;
        tc2=t;
    end
%% Run estimators of gamma
    gamma_c_hat=gamma_c0+vp*(t-tc2);
    gamma_c_n1_hat=gamma_cn1+vp*(t-tcn12);
    gamma_c_n2_hat=gamma_cn2+vp*(t-tcn22);
%% Accumulate error for integration term
    Ts=0.2;
    if (Re_Data1(2)~=0)                                                    % accumulate error when recieve new data from neigbor
       e=gamma_c_M-Re_Data1(2);
       e_int_t=e_int_t+.5*Ts*e;
    end
    if (Re_Data2(2)~=0) 
       e=gamma_c_M-Re_Data2(2);
       e_int_t=e_int_t+.5*Ts*e;
    end
%% Compute correction term 
    kg=.1;
    ki=.000;
    e1=(gamma_c_M-0.5*(gamma_c_n1_hat+gamma_c_n2_hat));
%     e1=(gamma_c_M-0.5*(Re_Data1(2)+Re_Data2(2)));
    vd_t=-kg*e1-ki*e_int_t;
    vd_t_max=vp;
    vd_t_min=-vp;
    if  vd_t<vd_t_min;
        vd_t=vd_t_min;
    elseif vd_t>=vd_t_max
        vd_t=vd_t_max;
    end
%% Prepare Data for transmition block
    gamma_e=gamma_c-gamma_c_hat;
    DataToTran=[gamma_c;gamma_e];
end
%% Path
function [gamma_c,pd,pd_gamma,vd_bar] = path(gamma,vp,L,R,d,m) 
s1=L-m;
s2=s1+pi*(R-d);
s3=s2+L;
s4=s3+pi*(R+d);
s5=s4+m;
ratio1=(R-d)/R;
ratio2=(R+d)/R;
% ratio1=1;
% ratio2=1;
 
if gamma<s5;
    cycle=0;
else
    cycle=1;
end
s=gamma-s5*cycle;
if s<s1                                    % first segment of straight line;
    vd_bar=vp;
    xd=s+R+m;
    yd=0+d;
    pd_gamma=[1;0];      
    gamma_c=s+s5*cycle;                                  % the segment is parallel with x
elseif (s>=s1) && (s<=s2)                  % second segment, a circumference 
    vd_bar=ratio1*vp;
    psi_T=(s-s1)/(R-d);
    xd=L+R+(R-d)*sin(psi_T);   
    yd=d+(R-d)*(1-cos(psi_T));
    pd_gamma=[cos(psi_T);sin(psi_T)];
    gamma_c=s1+(s-s1)*R/(R-d)+s5*cycle; 
elseif (s>s2) && (s<=s3)                   % third segment, a straight line 
    vd_bar=vp;
    xd=s3-s+R;  
    yd=d+2*(R-d); 
    pd_gamma=[-1;0];
    gamma_c=s+d*pi+s5*cycle;
elseif (s>s3) && (s<=s4)   
    vd_bar=ratio2*vp;
    xd=R-(R+d)*sin((s-s3)/(R+d));
    yd=d+2*(R-d)+(R+d)*(1-cos((s-s3)/(R+d)));
    pd_gamma=[-cos((s-s3)/(R+d));sin((s-s3)/(R+d))]; 
    gamma_c=s3+d*pi+(s-s3)*R/(R+d)+s5*cycle;   
else
    vd_bar=vp;
    xd=(s-s4)+R;
    yd=d+4*R;
    pd_gamma=[1;0];
    gamma_c=s+s5*cycle;
end
if cycle ==0
pd=[xd;cycle*4*R+yd];
else 
pd=[xd;cycle*4*R+yd];
end

end

== matlab function Simplified Estimator of Gamma for two vehicle1/Estimator ==
  data: vd_t output double size=1; DataToTran output double size=2; gamma_c input double; gamma_c_M input double; t input double; Re_Data1 input double size=2; Re_Data2 input double; Com_Sig input double; gamma_hat output double; tau_bar input double; Mode input double; vd input double; e_int input double; e output double; e_int_event output double
function [vd_t,DataToTran,gamma_hat,e,e_int_event] = fcn(gamma_c,gamma_c_M,t,Re_Data1,Re_Data2,Com_Sig,tau_bar,Mode,vd,e_int)

%% 
kg=1;
% L=[1 -1;
%    -1 1]; 

%% Reset estimator of gamma
persistent gamma_cn1 gamma_cn2 gamma_c0 tc1 tc2 tcn11 tcn12 tcn21 tcn22 tem_c tem_cn1 tem_cn2 reset_c reset_cn1 reset_cn2 e_int_t;   
if isempty(gamma_cn1)
    gamma_cn1=0;
    gamma_cn2=0;
    gamma_c0=0;
    tcn11=t;
    tcn12=t;
    tcn21=t;
    tcn22=t;
    tc1=t;
    tc2=t;
    tem_c=t;
    tem_cn1=t;
    tem_cn2=t;
    reset_c=false;
    reset_cn1=false;
    reset_cn2=false;
    e_int_t=0;
end
%% Reset estimator for gamma_c of first neighbor;
if (Re_Data1(1)~=0)                                  % If recived new data, reset estimator that the current vehicle thinks about the neighbor vehicle
    tcn11=Re_Data1(1); 
    tem_cn1=Re_Data1(2);
    reset_cn1=true;
end   
if (t-tcn11>tau_bar)&&reset_cn1
    gamma_cn1=tem_cn1+vd*tau_bar;
    reset_cn1=false;
    tcn12=t;
end
%% Reset estimator for gamma_c of second neighbor;
if (Re_Data2(1)~=0)                                  % If recived new data, reset estimator that the current vehicle thinks about the neighbor vehicle
    tcn21=Re_Data1(1); 
    tem_cn2=Re_Data2(2);
    reset_cn2=true;
end   
if (t-tcn21>tau_bar)&&reset_cn2
    gamma_cn2=tem_cn2+vd*tau_bar;
    reset_cn2=false;
    tcn22=t;
end
%% Reset estimator for gamma_c of current vehicle   % When it sends its coordinate state to neighbor, it needs to update its estimator too to synchoronize with the neighbor
if (Com_Sig~=0)
    tc1=t;
    tem_c=gamma_c;
    reset_c=true;
end
if (t-tc1>tau_bar)&& reset_c
    gamma_c0=tem_c+vd*tau_bar;
    reset_c=false;
    tc2=t;
end
%% Run estimators
gamma_c_hat=gamma_c0+vd*(t-tc2);
gamma_c_n1_hat=gamma_cn1+vd*(t-tcn12);
gamma_c_n2_hat=gamma_cn2+vd*(t-tcn22);

gamma_hat=[gamma_c_hat;gamma_c_n1_hat;gamma_c_n2_hat]; 

ki=.1;
if Mode==0
     e=gamma_c_M-0.5*(Re_Data1(2)+Re_Data2(2));
elseif Mode==1
    if (Re_Data1(2)~=0)
       e=gamma_c_M-0.5*(Re_Data1(2)+Re_Data2(2));
    else   
       e=0;
    end
else
    if (Re_Data1(2)~=0) 
       e=gamma_c_M-Re_Data1(2);
       e_int_t=e_int_t+e;
    else
        e=0;
    end
     if (Re_Data2(2)~=0) 
       e=gamma_c_M-Re_Data2(2);
       e_int_t=e_int_t+e;
     else
         e=0;
     end
end
%% Compute correction term 
if Mode==0;                                     % if Mode==0, continous communication, we use direct data recieved from neighbor.
    vd_t=-kg*e-ki*e_int; 
elseif Mode==1
    e1=(gamma_c-0.5*(gamma_c_n1_hat+gamma_c_n2_hat));
    vd_t=-kg*e1-ki*e_int;
else
    e1=(gamma_c-0.5*(gamma_c_n1_hat+gamma_c_n2_hat));
    vd_t=-kg*e1-ki*e_int_t;
end
e_int_event=e_int_t;
%% Prepare Data for transmition block
gamma_e=gamma_c-gamma_c_hat;
% DataToTran=[gamma_c;gamma_e;gamma_hat];
DataToTran=[gamma_c;gamma_e];
